simulink model "optimal2Area_Optimal"  (R2022a)
settings: Solver=ode23  StartTime=0.0  StopTime=60  MaxStep=1e-3  RelTol=1e-3
values from neighbouring files (symbols this model uses):
  A = [ ... (first row only)    [Ricatti_CallForOptimal.m]
  B = BT'    [Ricatti_CallForOptimal.m]
  b1 = 0.425    [CallForSingleArea.m]    (also in Ricatti_CallForOptimal.m)
  CT = [ ... (first row only)    [Ricatti_CallForOptimal.m]
  F = FT'    [Ricatti_CallForOptimal.m]
  Z = [z1;z2]    [Ricatti_CallForOptimal.m]
undefined symbols (not defined in the file or in its folder): K
settings Model: Creator=ASUS  LastModifiedBy=ASUS

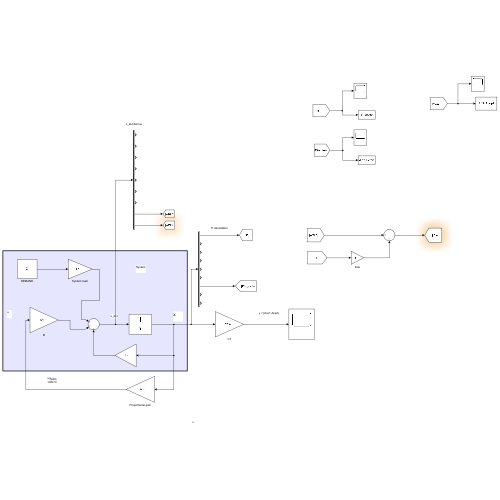
[thumbnail: Simulink's stored preview of the top-level diagram]
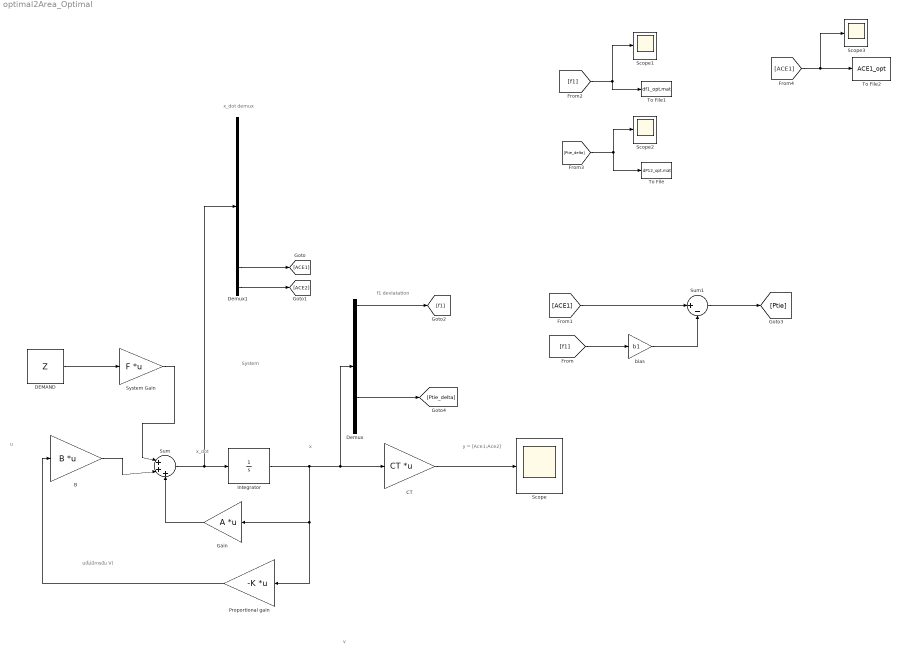
== system optimal2Area_Optimal ==
  note: x_dot demux
  note: System
  note: f1 deviatation
  note: u(ไม่มีการปัน V)
  note: y = [Ace1;Ace2]
  note: u
  note: x_dot
  note: x
  note: v
  B : Gain  Gain=B  Multiplication=Matrix(K*u)
  CT : Gain  Gain=CT  Multiplication=Matrix(K*u)
  DEMAND : Constant  Value=Z
  Demux : Demux  Outputs=9
  Demux1 : Demux  Outputs=9
  Gain : Gain  Gain=A  Multiplication=Matrix(K*u)
  Integrator : Integrator
  Proportional gain : Gain  Gain=-K  Multiplication=Matrix(K*u)
  Scope{,1..3} (4 alike) : Scope
  Sum : Sum  Inputs=|+++
  Sum1 : Sum  Inputs=|+-
  System Gain : Gain  Gain=F  Multiplication=Matrix(K*u)
  To File : ToFile  Filename=dP12_opt.mat  MatrixName=dP12_opt
  To File1 : ToFile  Filename=df1_opt.mat  MatrixName=df1_opt
  To File2 : ToFile  Filename=ACE1_opt  MatrixName=ACE1_opt  SaveFormat=Timeseries
  bias : Gain  Gain=b1
  wires:
  DEMAND/1 -> System Gain/1
  System Gain/1 -> Sum/1
  B/1 -> Sum/2
  Sum/1 -> Demux1/1, Integrator/1
  Integrator/1 -> Gain/1, Proportional gain/1, Demux/1, CT/1
  CT/1 -> Scope/1
  Demux/1 -> [f1]
  Proportional gain/1 -> B/1
  Gain/1 -> Sum/3
  Demux1/8 -> [ACE1]
  Demux1/9 -> [ACE2]
  [ACE1] -> Sum1/1
  [f1] -> bias/1
  bias/1 -> Sum1/2
  Sum1/1 -> [Ptie]
  [f1] -> To File1/1, Scope1/1
  [Ptie_delta] -> To File/1, Scope2/1
  Demux/7 -> [Ptie_delta]
  [ACE1] -> To File2/1, Scope3/1
